simulink model "Semi_DP_1Hz"  (Simulink 8.7)
settings: Solver=ode4  StartTime=0.0  StopTime=12600  FixedStep=1  RelTol=1e-3
PreLoadFcn:
  | load('Initialization_data.mat');
undefined symbols (not defined in the file or in its folder): D, M, Ma, magnitude, P_mean, QTF_Dir, QTF_Freq, QTF_P, QTF_P1, QTF_Phase, QTF_T, RAO_Amp, RAO_Dir, RAO_Freq, RAO_Phase, RAO_Vel
libraries: simulink_extras x5, simulink x3
(part 2 of 2)

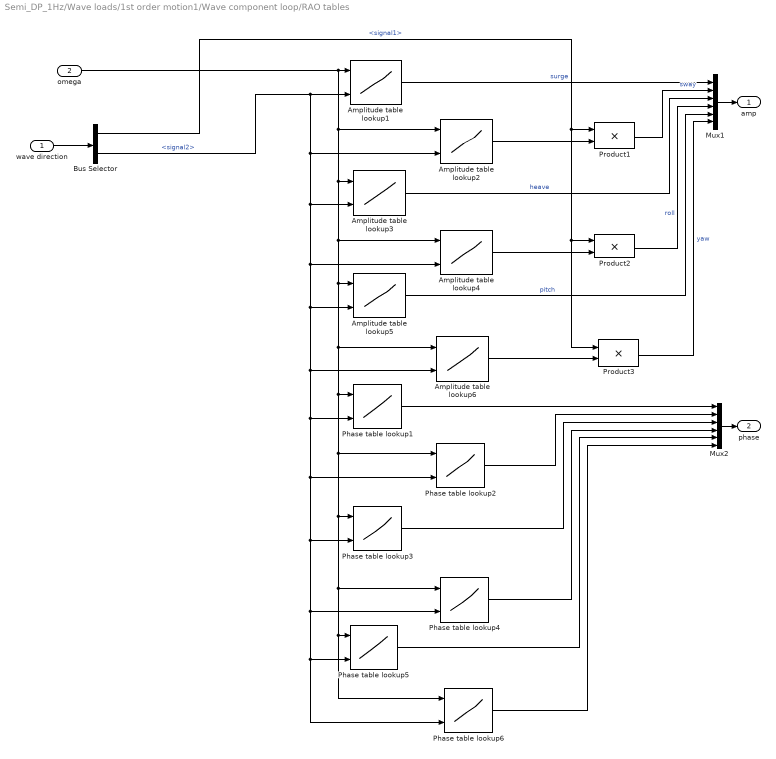
== system Semi_DP_1Hz/Wave loads/1st order motion1/Wave component loop/RAO tables ==
  wave direction : Inport
  omega : Inport  Port=2
  Amplitude table lookup1 : Lookup_n-D  BreakpointsForDimension1=RAO_Freq  BreakpointsForDimension2=RAO_Dir  BreakpointsForDimension3=RAO_Vel  Table=RAO_Amp(:,:,1)  DiagnosticForOutOfRangeInput=Warning  InputSameDT=on
  Amplitude table lookup2 : Lookup_n-D  BreakpointsForDimension1=RAO_Freq  BreakpointsForDimension2=RAO_Dir  BreakpointsForDimension3=RAO_Vel  Table=RAO_Amp(:,:,2)  InputSameDT=on
  Amplitude table lookup3 : Lookup_n-D  BreakpointsForDimension1=RAO_Freq  BreakpointsForDimension2=RAO_Dir  BreakpointsForDimension3=RAO_Vel  Table=RAO_Amp(:,:,3)  InputSameDT=on
  Amplitude table lookup4 : Lookup_n-D  BreakpointsForDimension1=RAO_Freq  BreakpointsForDimension2=RAO_Dir  BreakpointsForDimension3=RAO_Vel  Table=RAO_Amp(:,:,4)  InputSameDT=on
  Amplitude table lookup5 : Lookup_n-D  BreakpointsForDimension1=RAO_Freq  BreakpointsForDimension2=RAO_Dir  BreakpointsForDimension3=RAO_Vel  Table=RAO_Amp(:,:,5)  InputSameDT=on
  Amplitude table lookup6 : Lookup_n-D  BreakpointsForDimension1=RAO_Freq  BreakpointsForDimension2=RAO_Dir  BreakpointsForDimension3=RAO_Vel  Table=RAO_Amp(:,:,6)  InputSameDT=on
  Bus Selector : BusSelector  OutputSignals=signal1,signal2
  Mux1 : Mux  Inputs=6
  Mux2 : Mux  Inputs=6
  Phase table lookup1 : Lookup_n-D  BreakpointsForDimension1=RAO_Freq  BreakpointsForDimension2=RAO_Dir  BreakpointsForDimension3=RAO_Vel  Table=RAO_Phase(:,:,1)  InputSameDT=on
  Phase table lookup2 : Lookup_n-D  BreakpointsForDimension1=RAO_Freq  BreakpointsForDimension2=RAO_Dir  BreakpointsForDimension3=RAO_Vel  Table=RAO_Phase(:,:,2)  InputSameDT=on
  Phase table lookup3 : Lookup_n-D  BreakpointsForDimension1=RAO_Freq  BreakpointsForDimension2=RAO_Dir  BreakpointsForDimension3=RAO_Vel  Table=RAO_Phase(:,:,3)  InputSameDT=on
  Phase table lookup4 : Lookup_n-D  BreakpointsForDimension1=RAO_Freq  BreakpointsForDimension2=RAO_Dir  BreakpointsForDimension3=RAO_Vel  Table=RAO_Phase(:,:,4)  InputSameDT=on
  Phase table lookup5 : Lookup_n-D  BreakpointsForDimension1=RAO_Freq  BreakpointsForDimension2=RAO_Dir  BreakpointsForDimension3=RAO_Vel  Table=RAO_Phase(:,:,5)  InputSameDT=on
  Phase table lookup6 : Lookup_n-D  BreakpointsForDimension1=RAO_Freq  BreakpointsForDimension2=RAO_Dir  BreakpointsForDimension3=RAO_Vel  Table=RAO_Phase(:,:,6)  InputSameDT=on
  Product1 : Product  Inputs=**  SaturateOnIntegerOverflow=on  OutDataTypeStr=Inherit: Same as first input
  Product2 : Product  Inputs=**  SaturateOnIntegerOverflow=on  OutDataTypeStr=Inherit: Same as first input
  Product3 : Product  Inputs=**  SaturateOnIntegerOverflow=on  OutDataTypeStr=Inherit: Same as first input
  amp : Outport
  phase : Outport  Port=2
  wires:
  Product2/1 -> Mux1/4  "roll"
  Bus Selector/1 -> Product3/1, Product2/1, Product1/1  "<signal1>"
  Bus Selector/2 -> Amplitude table lookup1/2, Phase table lookup1/2, Phase table lookup5/2, Phase table lookup6/2, Phase table lookup4/2, Phase table lookup3/2, Phase table lookup2/2, Amplitude table lookup6/2, Amplitude table lookup5/2, Amplitude table lookup4/2, Amplitude table lookup3/2, Amplitude table lookup2/2  "<signal2>"
  wave direction/1 -> Bus Selector/1
  Amplitude table lookup1/1 -> Mux1/1  "surge"
  omega/1 -> Amplitude table lookup1/1, Phase table lookup1/1, Phase table lookup5/1, Phase table lookup6/1, Phase table lookup4/1, Phase table lookup3/1, Phase table lookup2/1, Amplitude table lookup6/1, Amplitude table lookup5/1, Amplitude table lookup4/1, Amplitude table lookup3/1, Amplitude table lookup2/1
  Amplitude table lookup3/1 -> Mux1/3  "heave"
  Amplitude table lookup5/1 -> Mux1/5  "pitch"
  Product1/1 -> Mux1/2  "sway"
  Amplitude table lookup2/1 -> Product1/2
  Amplitude table lookup4/1 -> Product2/2
  Product3/1 -> Mux1/6  "yaw"
  Amplitude table lookup6/1 -> Product3/2
  Mux2/1 -> phase/1
  Phase table lookup1/1 -> Mux2/1
  Phase table lookup2/1 -> Mux2/2
  Phase table lookup3/1 -> Mux2/3
  Phase table lookup4/1 -> Mux2/4
  Phase table lookup5/1 -> Mux2/5
  Phase table lookup6/1 -> Mux2/6
  Mux1/1 -> amp/1

== system Semi_DP_1Hz/Wave loads/Wave drift force (exact value)1/Wave component loop/calculation of theoredtical mean drift force ==
  Wave direction : Inport
  Omega : Inport  Port=2
  Zeta_a : Inport  Port=3
  number of  iterations : Inport  Port=4
  Constant1 : Constant  Value=2
  For Iterator : ForIterator  ResetStates=reset  IterationSource=external  IterationVariableDataType=double
  Math Function2 : Math  Operator=pow  SaturateOnIntegerOverflow=on
  Memory1 : Memory  InheritSampleTime=on
  Product2 : Product  RndMeth=Zero
  QTF tables1 : Subsystem
  Selector2 : Selector  IndexOptions=Index vector (port)  Indices=[1 3]  OutputSizes=1
  Selector4 : Selector  IndexOptions=Index vector (port)  Indices=[1 3]  OutputSizes=1
  Sum1 : Sum  Inputs=|++
  theoretical mean drift force : Outport
  wires:
  QTF tables1/1(mean drift force QTF_P) -> Product2/1
  Wave direction/1 -> QTF tables1/1(wave direction)
  Selector2/1 -> QTF tables1/2(omega)  "omega"
  number of  iterations/1 -> For Iterator/1
  Omega/1 -> Selector2/1
  For Iterator/1 -> Selector2/2, Selector4/2  "i=1:N"
  Zeta_a/1 -> Selector4/1
  Selector4/1 -> Math Function2/1
  Constant1/1 -> Math Function2/2
  Math Function2/1 -> Product2/2
  Memory1/1 -> Sum1/2
  Sum1/1 -> Memory1/1, theoretical mean drift force/1
  Product2/1 -> Sum1/1

== system Semi_DP_1Hz/Wave loads/Wave drift force (exact value)1/Wave component loop/calculation of theoretical slowly varying drift force ==
  number of  iterations : Inport
  Wave direction : Inport  Port=2
  Omega : Inport  Port=3
  Zeta_a : Inport  Port=4
  Phase_total : Inport  Port=5
  Add : Sum  Inputs=-+
  For Iterator : ForIterator  ResetStates=reset  IterationSource=external  IterationVariableDataType=double
  Memory : Memory  InheritSampleTime=on
  Selector2 : Selector  IndexOptions=Index vector (port)  Indices=[1 3]  OutputSizes=1
  Selector3 : Selector  IndexOptions=Index vector (port)  Indices=[1 3]  OutputSizes=1
  Selector4 : Selector  IndexOptions=Index vector (port)  Indices=[1 3]  OutputSizes=1
  Sum : Sum  Inputs=|++
  j loop : Subsystem  TreatAsAtomicUnit=on
  theoretical S_V drift force : Outport
  wires:
  Add/1 -> j loop/9(number of iterations)
  j loop/1(j loop) -> Sum/1
  Sum/1 -> theoretical S_V drift force/1, Memory/1
  Memory/1 -> Sum/2
  Selector3/1 -> j loop/5(Phase(i))  "phase"
  Phase_total/1 -> j loop/4(Phase), Selector3/1
  Omega/1 -> j loop/2(Omega), Selector2/1
  Wave direction/1 -> j loop/1(Wave direction)
  Selector4/1 -> j loop/7(Zeta_a(i))
  Zeta_a/1 -> j loop/6(Zeta_a), Selector4/1
  For Iterator/1 -> Add/1, j loop/8(i loop), Selector3/2, Selector2/2, Selector4/2  "i=1:N"
  number of  iterations/1 -> Add/2, For Iterator/1
  Selector2/1 -> j loop/3(Omega(i))  "omega"

== system Semi_DP_1Hz/Wave loads/Wave drift force (exact value)1/Wave component loop/calculation of theoredtical mean drift force/QTF tables1 ==
  wave direction : Inport
  omega : Inport  Port=2
  Mux1 : Mux  Inputs=3
  Mux2 : Mux  Inputs=3
  QTF table lookup1 : Lookup_n-D  BreakpointsForDimension1=QTF_Freq  BreakpointsForDimension2=QTF_Dir  BreakpointsForDimension3=RAO_Vel  Table=QTF_P(:,:,1)  DiagnosticForOutOfRangeInput=Warning  InputSameDT=on
  QTF table lookup2 : Lookup_n-D  BreakpointsForDimension1=QTF_Freq  BreakpointsForDimension2=QTF_Dir  BreakpointsForDimension3=RAO_Vel  Table=QTF_P(:,:,2)  InputSameDT=on
  QTF table lookup3 : Lookup_n-D  BreakpointsForDimension1=QTF_Freq  BreakpointsForDimension2=QTF_Dir  BreakpointsForDimension3=RAO_Vel  Table=QTF_P(:,:,3)  InputSameDT=on
  QTF table lookup4 : Lookup_n-D  BreakpointsForDimension1=QTF_Freq  BreakpointsForDimension2=QTF_Dir  BreakpointsForDimension3=RAO_Vel  Table=QTF_P(:,:,4)  InputSameDT=on
  QTF table lookup5 : Lookup_n-D  BreakpointsForDimension1=QTF_Freq  BreakpointsForDimension2=QTF_Dir  BreakpointsForDimension3=RAO_Vel  Table=QTF_P(:,:,5)  InputSameDT=on
  QTF table lookup6 : Lookup_n-D  BreakpointsForDimension1=QTF_Freq  BreakpointsForDimension2=QTF_Dir  BreakpointsForDimension3=RAO_Vel  Table=QTF_P1(:,:,6)  InputSameDT=on
  Terminator : Terminator
  mean drift force QTF_P : Outport
  wires:
  Mux2/1 -> Terminator/1
  QTF table lookup5/1 -> Mux2/3  "pitch"
  QTF table lookup4/1 -> Mux2/2  "roll"
  QTF table lookup3/1 -> Mux2/1  "heave"
  QTF table lookup1/1 -> Mux1/1  "surge"
  QTF table lookup2/1 -> Mux1/2  "sway"
  Mux1/1 -> mean drift force QTF_P/1
  QTF table lookup6/1 -> Mux1/3  "yaw"
  omega/1 -> QTF table lookup2/1, QTF table lookup3/1, QTF table lookup4/1, QTF table lookup6/1, QTF table lookup5/1, QTF table lookup1/1
  wave direction/1 -> QTF table lookup2/2, QTF table lookup3/2, QTF table lookup4/2, QTF table lookup6/2, QTF table lookup5/2, QTF table lookup1/2

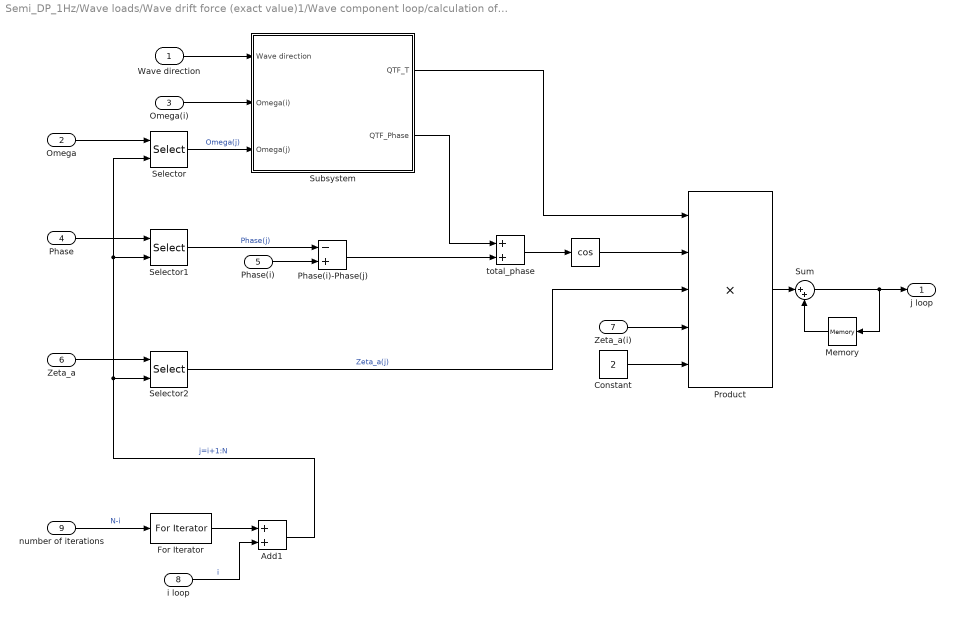
== system Semi_DP_1Hz/Wave loads/Wave drift force (exact value)1/Wave component loop/calculation of theoretical slowly varying drift force/j loop ==
  Wave direction : Inport
  Omega : Inport  Port=2
  Omega(i) : Inport  Port=3
  Phase : Inport  Port=4
  Phase(i) : Inport  Port=5
  Zeta_a : Inport  Port=6
  Zeta_a(i) : Inport  Port=7
  i loop : Inport  Port=8
  number of iterations : Inport  Port=9
  " " : Trigonometry  Operator=cos
  Add1 : Sum
  Constant : Constant  Value=2
  For Iterator : ForIterator  ResetStates=reset  IterationSource=external  IterationVariableDataType=double
  Memory : Memory  InheritSampleTime=on
  Phase(i)-Phase(j) : Sum  Inputs=-+
  Product : Product  Inputs=5  RndMeth=Zero
  Selector : Selector  IndexOptions=Index vector (port)  Indices=[1 3]  OutputSizes=1
  Selector1 : Selector  IndexOptions=Index vector (port)  Indices=[1 3]  OutputSizes=1
  Selector2 : Selector  IndexOptions=Index vector (port)  Indices=[1 3]  OutputSizes=1
  Subsystem : Subsystem
  Sum : Sum  Inputs=|++
  total_phase : Sum
  j loop : Outport
  wires:
  number of iterations/1 -> For Iterator/1  "N-i"
  Product/1 -> Sum/1
  Sum/1 -> j loop/1, Memory/1
  Memory/1 -> Sum/2
  Constant/1 -> Product/5
  Zeta_a(i)/1 -> Product/4
  Selector2/1 -> Product/3  "Zeta_a(j)"
  " "/1 -> Product/2
  Subsystem/1(QTF_T) -> Product/1
  total_phase/1 -> " "/1
  Subsystem/2(QTF_Phase) -> total_phase/1
  Phase(i)-Phase(j)/1 -> total_phase/2
  Phase(i)/1 -> Phase(i)-Phase(j)/2
  Selector1/1 -> Phase(i)-Phase(j)/1  "Phase(j)"
  Add1/1 -> Selector/2, Selector1/2, Selector2/2  "j=i+1:N"
  For Iterator/1 -> Add1/1
  i loop/1 -> Add1/2  "i"
  Zeta_a/1 -> Selector2/1
  Phase/1 -> Selector1/1
  Selector/1 -> Subsystem/3(Omega(j))  "Omega(j)"
  Omega(i)/1 -> Subsystem/2(Omega(i))
  Wave direction/1 -> Subsystem/1(Wave direction)
  Omega/1 -> Selector/1

== system Semi_DP_1Hz/Wave loads/Wave drift force (exact value)1/Wave component loop/calculation of theoretical slowly varying drift force/j loop/Subsystem ==
  Wave direction : Inport
  Omega(i) : Inport  Port=2
  Omega(j) : Inport  Port=3
  Mux : Mux  Inputs=3
  Mux1 : Mux  Inputs=3
  n-D Lookup Table : Lookup_n-D  NumberOfTableDimensions=3  BreakpointsForDimension1=QTF_Freq  BreakpointsForDimension2=QTF_Freq  BreakpointsForDimension3=QTF_Dir  Table=QTF_T(:,:,:,1)  ExtrapMethod=Clip  UseLastTableValue=on  RndMeth=Simplest  InputSameDT=on
  n-D Lookup Table1 : Lookup_n-D  NumberOfTableDimensions=3  BreakpointsForDimension1=QTF_Freq  BreakpointsForDimension2=QTF_Freq  BreakpointsForDimension3=QTF_Dir  Table=QTF_Phase(:,:,:,1)  ExtrapMethod=Clip  UseLastTableValue=on  RndMeth=Simplest  InputSameDT=on
  n-D Lookup Table2 : Lookup_n-D  NumberOfTableDimensions=3  BreakpointsForDimension1=QTF_Freq  BreakpointsForDimension2=QTF_Freq  BreakpointsForDimension3=QTF_Dir  Table=QTF_T(:,:,:,2)  ExtrapMethod=Clip  UseLastTableValue=on  RndMeth=Simplest  InputSameDT=on
  n-D Lookup Table3 : Lookup_n-D  NumberOfTableDimensions=3  BreakpointsForDimension1=QTF_Freq  BreakpointsForDimension2=QTF_Freq  BreakpointsForDimension3=QTF_Dir  Table=QTF_Phase(:,:,:,2)  ExtrapMethod=Clip  UseLastTableValue=on  RndMeth=Simplest  InputSameDT=on
  n-D Lookup Table4 : Lookup_n-D  NumberOfTableDimensions=3  BreakpointsForDimension1=QTF_Freq  BreakpointsForDimension2=QTF_Freq  BreakpointsForDimension3=QTF_Dir  Table=QTF_T(:,:,:,6)  ExtrapMethod=Clip  UseLastTableValue=on  RndMeth=Simplest  InputSameDT=on
  n-D Lookup Table5 : Lookup_n-D  NumberOfTableDimensions=3  BreakpointsForDimension1=QTF_Freq  BreakpointsForDimension2=QTF_Freq  BreakpointsForDimension3=QTF_Dir  Table=QTF_Phase(:,:,:,6)  ExtrapMethod=Clip  UseLastTableValue=on  RndMeth=Simplest  InputSameDT=on
  QTF_T : Outport
  QTF_Phase : Outport  Port=2
  wires:
  Mux1/1 -> QTF_Phase/1
  Mux/1 -> QTF_T/1
  n-D Lookup Table5/1 -> Mux1/3
  n-D Lookup Table/1 -> Mux/1
  Wave direction/1 -> n-D Lookup Table2/3, n-D Lookup Table3/3, n-D Lookup Table5/3, n-D Lookup Table4/3, n-D Lookup Table1/3, n-D Lookup Table/3
  Omega(j)/1 -> n-D Lookup Table2/2, n-D Lookup Table3/2, n-D Lookup Table5/2, n-D Lookup Table4/2, n-D Lookup Table1/2, n-D Lookup Table/2
  Omega(i)/1 -> n-D Lookup Table5/1, n-D Lookup Table4/1, n-D Lookup Table3/1, n-D Lookup Table2/1, n-D Lookup Table/1, n-D Lookup Table1/1
  n-D Lookup Table4/1 -> Mux/3
  n-D Lookup Table3/1 -> Mux1/2
  n-D Lookup Table2/1 -> Mux/2
  n-D Lookup Table1/1 -> Mux1/1
